simulink model "quadcopter"  (R2020b)
settings: Solver=VariableStepAuto  StartTime=0.0  StopTime=10.0  RelTol=1e-6
undefined symbols (not defined in the file): b, d, g, Jr, Jx, Jy, Jz, L, m, q0, q1, q2, q3, vx, vy, vz, wx, wy, wz, x, y, z
settings Model: Creator=Amir  LastModifiedBy=Amir
settings DataIOCC: ReturnWorkspaceOutputs=off

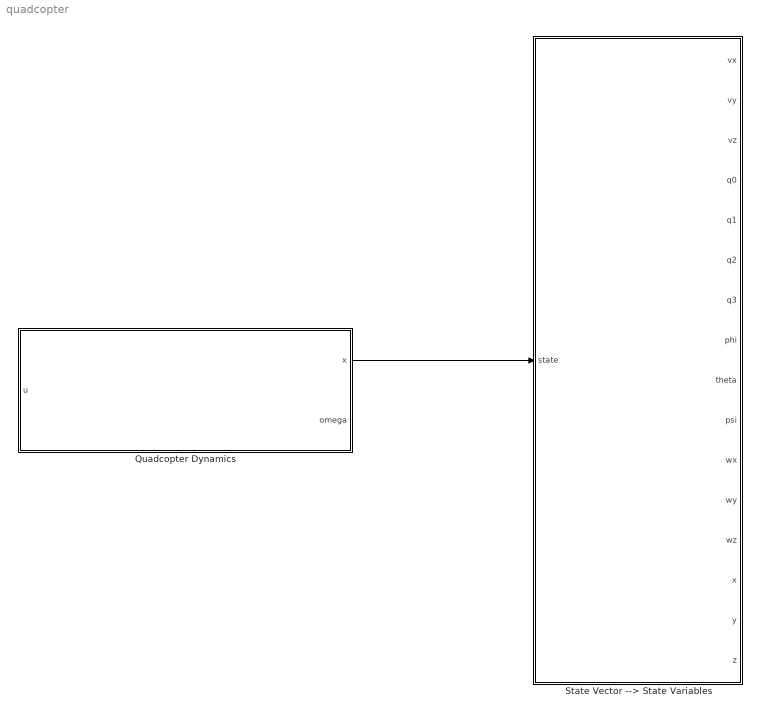
== system quadcopter ==
  Quadcopter Dynamics : Subsystem  mask(6DOF Quadcopter Dynamics Model){m=m, L=L, Jx=Jx, Jy=Jy, Jz=Jz, Jr=Jr, d=d, b=b, g=g, q=[q0;q1;q2;q3], w=[wx;wy;wz], xx=[x;y;z], v=[vx;vy;vz]}
      mask prompts: m "Quadcopter mass (m):"; L "Lever length (L):"; Jx "Quadcopter roll inertia (Jx):"; Jy "Quadcopter pitch inertia (Jy):"; Jz "Quadcopter yaw inertia (Jz):"; Jr "Rotor inertia (Jr):"; d "Drag factor (d):"; b "Thrust factor (b):"; g "gravity constant (g):"; q "Initial quaternion ([q0;q1;q2;q3]):"; w "Initial angular velocity ([wx;wy;wz]):"; xx "Initial position ([x;y;z]):"; v "Initial translational velocity ([vx;vy;vz]):"
      mask Help: The attitude of the quadcopter is modeled via quaternions. The state vector is constructed as X=[vx;vy;vz;;q0;q1;q2;q3;wx;wy;wz;x;y;z], where vx, vy, and vz stand for velocity elements, wx, wy, and wz stand for angular velocity elements, and x, y, and z stand for the position elements in each direction. Parameters q0, q1, q2, and q3 stand for quaternion entries.
      mask DialogControl DescGroupVar Prompt: Main
      mask DialogControl DescTextVar Prompt: Six degrees-of-freedom (6DOF) quadcopter dynamics model. Press the help button to see more details.
      mask DialogControl ParameterGroupVar_copy Prompt: Initial Conditions
      mask Display:
      | image('$imagefile'); % Use "Edit Image" on toolstrip to change.
      | color('red'); port_label('output',1,'State Vector (X)')
      | port_label('output',2,'Rotors Speed (Omega)')
      | port_label('input',1,'Control Input (U)')
  State Vector --> State Variables : MATLAB Function  TreatAsAtomicUnit=on
  wires:
  Quadcopter Dynamics/1(x) -> State Vector --> State Variables/1(state)

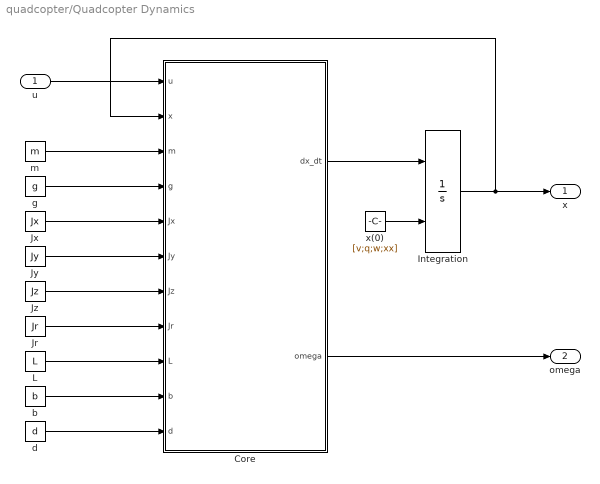
== system quadcopter/Quadcopter Dynamics ==
  u : Inport
  Core : MATLAB Function  TreatAsAtomicUnit=on
  Integration : Integrator  InitialConditionSource=external
  Jr : Constant  Value=Jr
  Jx : Constant  Value=Jx
  Jy : Constant  Value=Jy
  Jz : Constant  Value=Jz
  L : Constant  Value=L
  b : Constant  Value=b
  d : Constant  Value=d
  g : Constant  Value=g
  m : Constant  Value=m
  x(0) : Constant  Value=[v;q;w;xx]
  x : Outport
  omega : Outport  Port=2
  wires:
  Core/1(dx_dt) -> Integration/1
  x(0)/1 -> Integration/2
  Integration/1 -> x/1, Core/2(x)
  u/1 -> Core/1(u)
  m/1 -> Core/3(m)
  g/1 -> Core/4(g)
  Jx/1 -> Core/5(Jx)
  Jy/1 -> Core/6(Jy)
  Jz/1 -> Core/7(Jz)
  Jr/1 -> Core/8(Jr)
  L/1 -> Core/9(L)
  b/1 -> Core/10(b)
  d/1 -> Core/11(d)
  Core/2(omega) -> omega/1

== matlab function quadcopter/State Vector --> State Variables ==
  data: vx output; vy output; vz output; q0 output; q1 output; q2 output; q3 output; phi output; theta output; psi output; wx output; wy output; wz output; x output; state input size=[13 1]; y output; z output
function [vx,vy,vz,q0,q1,q2,q3,phi,theta,psi,wx,wy,wz,x,y,z] = demux(state)

vx = state(1);
vy = state(2);
vz = state(3);
q0 = state(4);
q1 = state(5);
q2 = state(6);
q3 = state(7);
wx = state(8);
wy = state(9);
wz = state(10);
x = state(11);
y = state(12);
z = state(13);


eulang = [atan2(2*(q2*q3+q0*q1),q0^2-q1^2-q2^2+q3^2)
         -asin(2*(q1*q3-q0*q2))
          atan2(2*(q1*q2+q0*q3),q0^2+q1^2-q2^2-q3^2)];
    
phi   = eulang(1);
theta = eulang(2);
psi   = eulang(3);

== matlab function quadcopter/Quadcopter Dynamics/Core ==
  data: u input size=[4 1]; dx_dt output size=[13 1]; x input size=[13 1]; m input; g input; Jx input; Jy input; Jz input; Jr input; L input; b input; d input; omega output
function [dx_dt,omega]  = quad_dyn(u,x,m,g,Jx,Jy,Jz,Jr,L,b,d)

BD=[b  b  b  b
    0  b  0 -b
    b  0 -b  0
    d -d  d -d];

% u=BD*omega.^2;

omega=(BD\u).^0.5;

% invBD=inv(BD);

% omega_u1=0.5*[invBD(1,1)
%               invBD(2,1)
%               invBD(3,1)
%               invBD(4,1)].*(BD\u).^(-0.5);
%           
% omega_u2=0.5*[invBD(1,2)
%               invBD(2,2)
%               invBD(3,2)
%               invBD(4,2)].*(BD\u).^(-0.5);
%           
% omega_u3=0.5*[invBD(1,3)
%               invBD(2,3)
%               invBD(3,3)
%               invBD(4,3)].*(BD\u).^(-0.5);
%           
% omega_u4=0.5*[invBD(1,4)
%               invBD(2,4)
%               invBD(3,4)
%               invBD(4,4)].*(BD\u).^(-0.5);

gu=omega(1)-omega(2)+omega(3)-omega(4);

% gu_u1=omega_u1(1)-omega_u1(2)+omega_u1(3)-omega_u1(4);
% gu_u2=omega_u2(1)-omega_u2(2)+omega_u2(3)-omega_u2(4);
% gu_u3=omega_u3(1)-omega_u3(2)+omega_u3(3)-omega_u3(4);
% gu_u4=omega_u4(1)-omega_u4(2)+omega_u4(3)-omega_u4(4);

dx_dt = [-2*(x(5)*x(7)+x(4)*x(6))*u(1)/m
         -2*(x(6)*x(7)-x(4)*x(5))*u(1)/m
          g-(x(4)^2-x(5)^2-x(6)^2+x(7)^2)*u(1)/m
          0.5*(-x(5)*x(8)-x(6)*x(9)-x(7)*x(10))
          0.5*(x(4)*x(8)-x(7)*x(9)+x(6)*x(10))
          0.5*(x(7)*x(8)+x(4)*x(9)-x(5)*x(10))
          0.5*(-x(6)*x(8)+x(5)*x(9)+x(4)*x(10))
          x(9)*x(10)*(Jy-Jz)/Jx-Jr/Jx*x(9)*gu+L/Jx*u(2)
          x(8)*x(10)*(Jz-Jx)/Jy+Jr/Jy*x(8)*gu+L/Jy*u(3)
          x(8)*x(9)*(Jx-Jy)/Jz+1/Jz*u(4)
          x(1)
          x(2)
          x(3)];

% A=[0 0 0 -2*x(6)*u(1)/m -2*x(7)*u(1)/m -2*x(4)*u(1)/m -2*x(5)*u(1)/m  0                          0                          0               0 0 0
%    0 0 0  2*x(5)*u(1)/m  2*x(4)*u(1)/m -2*x(7)*u(1)/m -2*x(6)*u(1)/m  0                          0                          0               0 0 0
%    0 0 0 -2*x(4)*u(1)/m  2*x(5)*u(1)/m  2*x(6)*u(1)/m -2*x(7)*u(1)/m  0                          0                          0               0 0 0
%    0 0 0  0             -0.5*x(8)      -0.5*x(9)      -0.5*x(10)     -0.5*x(5)                  -0.5*x(6)                  -0.5*x(7)        0 0 0
%    0 0 0  0.5*x(8)       0              0.5*x(10)     -0.5*x(9)       0.5*x(4)                  -0.5*x(7)                   0.5*x(6)        0 0 0
%    0 0 0  0.5*x(9)      -0.5*x(10)      0              0.5*x(8)       0.5*x(7)                   0.5*x(4)                  -0.5*x(5)        0 0 0
%    0 0 0  0.5*x(10)      0.5*x(9)      -0.5*x(8)       0             -0.5*x(6)                   0.5*x(5)                   0.5*x(4)        0 0 0
%    0 0 0  0              0              0              0              0                          x(10)*(Jy-Jz)/Jx-Jr/Jx*gu  x(9)*(Jy-Jz)/Jx 0 0 0
%    0 0 0  0              0              0              0              x(10)*(Jz-Jx)/Jy+Jr/Jy*gu  0                          x(8)*(Jz-Jx)/Jy 0 0 0
%    0 0 0  0              0              0              0              x(9)*(Jx-Jy)/Jz            x(8)*(Jx-Jy)/Jz            0               0 0 0
%    1 0 0  0              0              0              0              0                          0                          0               0 0 0
%    0 1 0  0              0              0              0              0                          0                          0               0 0 0
%    0 0 1  0              0              0              0              0                          0                          0               0 0 0];
% 
% B=[-2*(x(5)*x(7)+x(4)*x(6))/m        0                      0                      0
%    -2*(x(6)*x(7)-x(4)*x(5))/m        0                      0                      0
%    -(x(4)^2-x(5)^2-x(6)^2+x(7)^2)/m  0                      0                      0
%     0                                0                      0                      0
%     0                                0                      0                      0
%     0                                0                      0                      0
%     0                                0                      0                      0
%    -Jr/Jx*x(9)*gu_u1                -Jr/Jx*x(9)*gu_u2+L/Jx -Jr/Jx*x(9)*gu_u3      -Jr/Jx*x(9)*gu_u4
%     Jr/Jy*x(8)*gu_u1                 Jr/Jy*x(8)*gu_u2       Jr/Jy*x(8)*gu_u3+L/Jy  Jr/Jy*x(8)*gu_u4
%     0                                0                      0                      1/Jz
%     0                                0                      0                      0
%     0                                0                      0                      0
%     0                                0                      0                      0];
% 
% Avec=reshape(A,13*13,1);
% 
% Bvec=reshape(B,13*4,1);
